simulink model "Filter_Test"  (R2019b)
settings: Solver=VariableStepAuto  StartTime=0.0  StopTime=0.02  RelTol=1e-3
libraries: simulink_extras x3
settings Model: Creator=Shishir  LastModifiedBy=Shishir

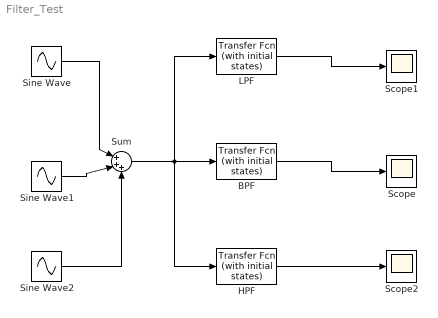
== system Filter_Test ==
  "BPF " : simulink_extras/Additional Linear/Transfer Fcn (with initial states)  N=[1.19E9 0 0]  D="[1  4.88E9 1.22E9 6.75E11 1.91E14]"  X0=0
  HPF : simulink_extras/Additional Linear/Transfer Fcn (with initial states)  N=[1 0 0]  D="[1  2.21E4 2.43E8]"  X0=0
  LPF : simulink_extras/Additional Linear/Transfer Fcn (with initial states)  N=[999200.16]  D="[1  1413.65 999200.16]"  X0=0
  Scope : Scope
  Scope1 : Scope
  Scope2 : Scope
  Sine Wave : Sin  Frequency=400  SampleTime=1/64000
  Sine Wave1 : Sin  Frequency=12000  SampleTime=1/64000
  Sine Wave2 : Sin  Frequency=31428.6  SampleTime=1/64000
  Sum : Sum  Inputs=|+++
  wires:
  Sum/1 -> HPF/1, "BPF "/1, LPF/1
  Sine Wave2/1 -> Sum/3
  Sine Wave1/1 -> Sum/2
  Sine Wave/1 -> Sum/1
  HPF/1 -> Scope2/1
  "BPF "/1 -> Scope/1
  LPF/1 -> Scope1/1
